simulink model "StateMachine_test"  (R2016a)
settings: Solver=FixedStepDiscrete  StartTime=0.0  StopTime=inf  FixedStep=0.001  RelTol=1e-3
PostLoadFcn:
  | build_location = fullfile(fileparts(which(bdroot)),'build');
  | 
  | set_param(0, 'CacheFolder', build_location);
  | set_param(0, 'CodeGenFolder', build_location);
InitFcn:
  | % Change dir to model location
  | cd(fileparts(which(bdroot)));
  | 
  | % Run init script
  | init_model;
  | 
  | load db.mat
  | initialize_model_param
StartFcn:
  | % Make sure we always move back to model folder
  | cd(fileparts(which(bdroot)));
StopFcn:
  | % Make sure we always move back to model folder
  | cd(fileparts(which(bdroot)));
model workspace (MAT data in the model file):
  localValue = 1
  targetValue = 0
libraries: xpcethercatlib x1, aerolibanimutils x1
CloseFcn:
  | % Make sure we always move back to model folder
  | cd(fileparts(which(bdroot)));
  | 
  | set_param(0, 'CacheFolder', '');
  | set_param(0, 'CodeGenFolder', '');
PauseFcn:
  | % Make sure we always move back to model folder
  | cd(fileparts(which(bdroot)));
ContinueFcn:
  | % Make sure we always move back to model folder
  | cd(fileparts(which(bdroot)));
settings Model: Creator=rtheyyun  LastModifiedBy=rafae
settings SolverCC: EnableConcurrentExecution=on  ConcurrentTasks=on
settings DataIOCC: LimitDataPoints=on  SaveFinalState=on  SaveFormat=StructureWithTime  SignalLoggingSaveFormat=ModelDataLogs  InspectSignalLogs=on
settings OptimizationCC: BlockReduction=off  OptimizeBlockIOStorage=off  BufferReuse=off  GlobalBufferReuse=off  ExpressionFolding=off  ExpressionDepthLimit=2147483647  LocalBlockOutputs=off
settings DebuggingCC: ReadBeforeWriteMsg=DisableAll  WriteAfterWriteMsg=DisableAll  WriteAfterReadMsg=DisableAll  UnderspecifiedInitializationDetection=Classic  MergeDetectMultiDrivingBlocksExec=none  SolverPrmCheckMsg=warning  InheritedTsInSrcMsg=none  FcnCallInpInsideContextMsg=UseLocalSettings  AllowSymbolicDim=off  StateNameClashWarn=warning
settings HardwareCC: ProdBitPerPointer=32  ProdLargestAtomicFloat=None  ProdWordSize=32  ProdLongLongMode=on  ProdHWDeviceType=Generic->32-bit x86 compatible
settings ModelReferenceCC: UpdateModelReferenceTargets=Force  PropagateSignalLabelsOutOfModel=off
settings RTWCC: SystemTargetFile=slrt.tlc  TemplateMakefile=slrt_default_tmf  Description=Simulink Real-Time  RTWVerbose=off
settings TargetCC: CodeReplacementLibrary=XPC_BLAS  ParMdlRefBuildCompliant=on  ConcurrentExecutionCompliant=on  MatFileLogging=on  MATLABClassNameForMDSCustomization=xpcAperiodicCustomization
settings ConfigComp: CovModelRefEnable=Off  CovSFcnEnable=off

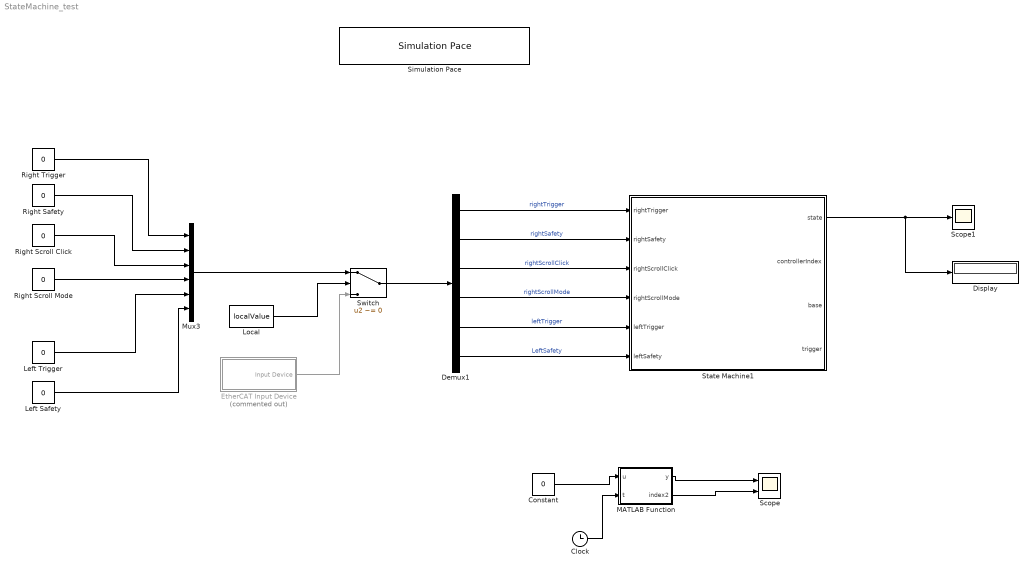
== system StateMachine_test ==
  Clock : Clock
  Constant : Constant  Value=0
  Demux1 : Demux  Outputs=6
  Display : Display
  EtherCAT Input Device : Subsystem  Commented=on
  Left Safety : Constant  Value=0
  Left Trigger : Constant  Value=0
  Local : Constant  Value=localValue
  MATLAB Function : MATLAB Function  TreatAsAtomicUnit=on
  Mux3 : Mux  Inputs=6
  Right Safety : Constant  Value=0
  Right Scroll Click : Constant  Value=0
  Right Scroll Mode : Constant  Value=0
  Right Trigger : Constant  Value=0
  Scope : Scope  NumInputPorts=2
  Scope1 : Scope
  Simulation Pace : aerolibanimutils/Simulation Pace  SimulationPace=1  SleepMode=MATLAB Thread  OutputPaceError=off  SampleTime=-1
  State Machine1 : Stateflow chart  TreatAsAtomicUnit=on
  Switch : Switch  Criteria=u2 ~= 0
  wires:
  Switch/1 -> Demux1/1
  Demux1/2 -> State Machine1/2(rightSafety)  "rightSafety"
  Demux1/3 -> State Machine1/3(rightScrollClick)  "rightScrollClick"
  Demux1/4 -> State Machine1/4(rightScrollMode)  "rightScrollMode"
  Demux1/5 -> State Machine1/5(leftTrigger)  "leftTrigger"
  Demux1/6 -> State Machine1/6(leftSafety)  "LeftSafety"
  Right Scroll Mode/1 -> Mux3/4
  Mux3/1 -> Switch/1
  Right Trigger/1 -> Mux3/1
  Right Safety/1 -> Mux3/2
  Right Scroll Click/1 -> Mux3/3
  Left Trigger/1 -> Mux3/5
  Local/1 -> Switch/2
  Left Safety/1 -> Mux3/6
  EtherCAT Input Device/1(Input Device) -> Switch/3
  Demux1/1 -> State Machine1/1(rightTrigger)  "rightTrigger"
  State Machine1/1(state) -> Display/1, Scope1/1
  Constant/1 -> MATLAB Function/1(u)
  MATLAB Function/1(y) -> Scope/1
  Clock/1 -> MATLAB Function/2(t)
  MATLAB Function/2(index2) -> Scope/2

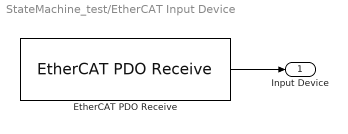
== system StateMachine_test/EtherCAT Input Device ==
  EtherCAT PDO Receive : xpcethercatlib/EtherCAT PDO Receive  Priority=2  sig_name=LHFE.Inputs.jointAngle  sig_offset=208  sig_type=uint32  type_size=32  sig_dim=1  device_id=0  sample_time=0.001000
  Input Device : Outport
  wires:
  EtherCAT PDO Receive/1 -> Input Device/1

== matlab function StateMachine_test/MATLAB Function ==
  data: u input; y output; t input; index2 output
function [y, index2] = fcn(u, t)

persistent index;

if t == 0
    index = 0;
end

if index == 1;
   a = t;
end


if u == 0;
    y = 0;
    index2 = 0;
else u == 1;
    y = 1;
    index = 1;
    index2 = index
end

== stateflow chart StateMachine_test/State Machine1 ==
  state Startup
    en: state = 0
    en: controllerIndex = 0
  state Sitting
    en: state = 1
    en: controllerIndex = 1
  state Standing
    en: state = 2
  state test
    en: controllerIndex = 2
    en: base = 3
    en: trigger = 4
  Sitting -> Startup [order 2] : [rightScrollMode == 0]
  (default) -> Startup : [rightScrollMode == 0]
  Startup -> Sitting : [rightScrollMode == 1]
  Standing -> Sitting : [rightScrollMode ==1]
  Sitting -> Standing [order 1] : [rightScrollMode == 2]
  data: rightTrigger input; rightSafety input; rightScrollClick input; rightScrollMode input; leftTrigger input; leftSafety input; state output; controllerIndex output; base output; trigger output
